simulink model "TB_submarine_mechanical"  (R2018b)
settings: Solver=VariableStepAuto  StartTime=0.0  StopTime=10.0  RelTol=1e-3
settings Model: Creator=Bruno Maric  LastModifiedBy=Bruno Maric

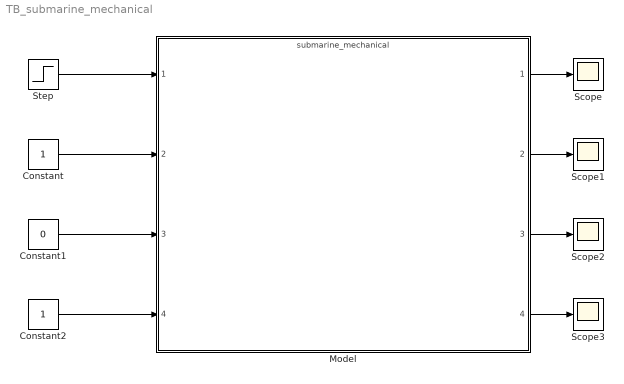
== system TB_submarine_mechanical ==
  Constant : Constant
  Constant1 : Constant  Value=0
  Constant2 : Constant
  Model : ModelReference  ModelNameDialog=submarine_mechanical.slx  SimulationMode=Normal  ModelReferenceVersion=1.27
  Scope{,1..3} (4 alike) : Scope
  Step : Step  Before=10  After=0  SampleTime=0
  wires:
  Step/1 -> Model/1
  Model/1 -> Scope/1
  Model/2 -> Scope1/1
  Model/3 -> Scope2/1
  Model/4 -> Scope3/1
  Constant/1 -> Model/2
  Constant1/1 -> Model/3
  Constant2/1 -> Model/4
